simulink model "test_current_limiter"  (R2025b)
settings: Solver=ode23  StartTime=0.0  StopTime=10.0  RelTol=1e-3
StopFcn:
  | Simulink.sdi.view;
  | Simulink.sdi.loadView('view_test_current_limiter');
libraries: fl_lib x6, nesl_utility x3, arsenal x1, ee_lib x1
settings Model: Creator=ggandolfi  LastModifiedBy=upattacini
settings DataIOCC: SaveOutput=off  DSMLogging=off  SaveTime=off  ReturnWorkspaceOutputs=off

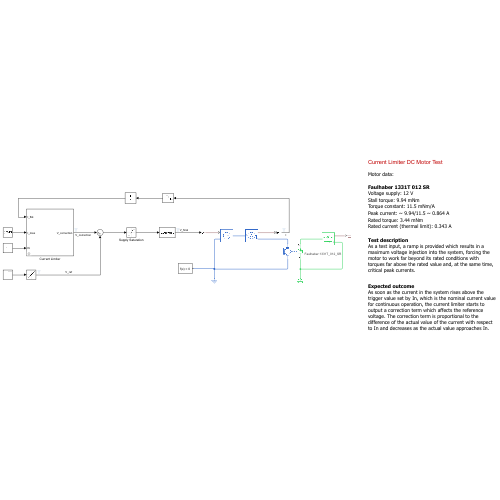
[thumbnail: Simulink's stored preview of the top-level diagram]
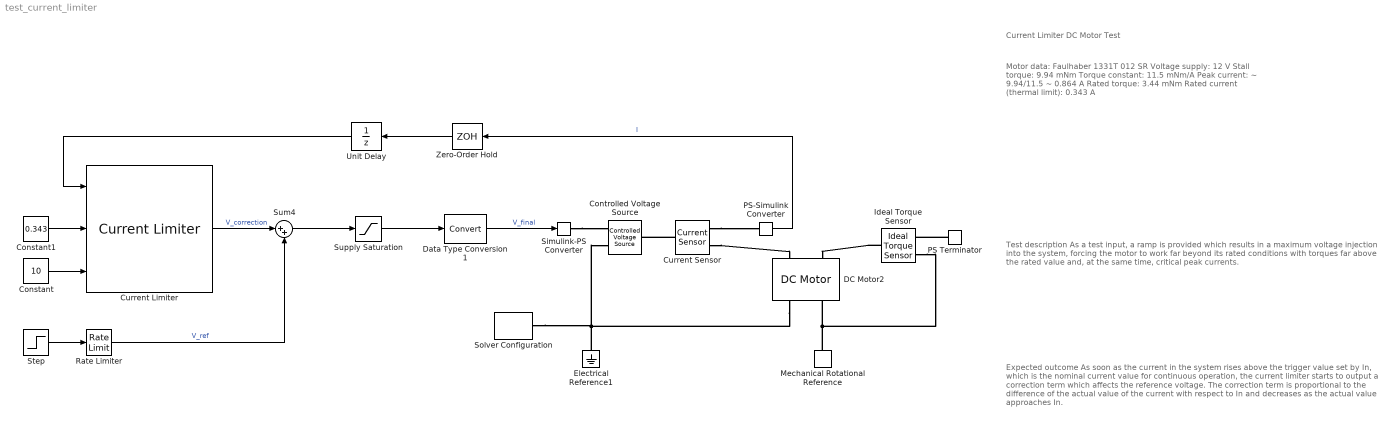
== system test_current_limiter ==
  note: Motor data:
      |
      | Faulhaber 1331T 012 SR
      | Voltage supply: 12 V
      | Stall torque: 9.94 mNm
      | Torque constant: 11.5 mNm/A
      | Peak current: ~ 9.94/11.5 ~ 0.864 A
      | Rated torque: 3.44 mNm
      | Rated current (thermal limit): 0.343 A
  note: Current Limiter DC Motor Test
  note: Test description
      | As a test input, a ramp is provided which results in a maximum voltage injection into the system, forcing the motor to work far beyond its rated conditions with torques far above the rated value and, at the same time, critical peak currents.
  note: Expected outcome
      | As soon as the current in the system rises above the trigger value set by In, which is the nominal current value for continuous operation, the current limiter starts to output a correction term which affects the reference voltage. The correction term is proportional to the difference of the actual value of the current with respect to In and decreases as the actual value approaches In.
  Constant : Constant  Value=10
  Constant1 : Constant  Value=0.343
  Controlled Voltage Source : fl_lib/Electrical/Electrical Sources/Controlled Voltage Source
  Current Limiter : arsenal/Signal Conditioning/Current Limiter  Ts=0.00005  I_max_gain=0.1  Discrete_time_integrator_gain=1.0
      settings: SourceProductName=MESH Arsenal
  Current Sensor : fl_lib/Electrical/Electrical Sensors/Current Sensor
  DC Motor2 : ee_lib/Electromechanical/Brushed Motors/DC Motor  PartSpecification="{\"CollectionId\":\"SimscapeElectrical\",\"DatasetId\":\"Faulhaber|1331T_012_SR|simscape.electrical.dcMotor\",\"DisplayName\":\"Faulhaber:1331T_012_SR\"}"  field_option=ee.enum.field_option.pm  Rf=100 % Parameter not set Ohm  Lf=1 % Parameter not set H  Laf=0.15 % Parameter not set H  If0=0 % Parameter not set A  parameterization=ee.enum.dcparam_option.torque_speed  Ra=13.7 % Datasheet derived Ohm  La=0.31 % Datasheet derived mH  emf_or_torque=ee.enum.emf_or_torque.ki  Kv=1.2 % Datasheet derived mV/rpm  Ki=11.5 % Parameter estimated mN*m/A  T_stall=9.94 m*mN  w_max=9910 rpm  w_rated=15000 % Parameter not set rpm  P_rated=0.08 % Parameter not set W  V_rated=10.5 V  lam_param=ee.enum.lam_param.current  i_noload=0.0105 % Datasheet derived A  V_i_noload=12 % Datasheet derived V  J=0.67 % Datasheet derived g*cm^2  lam=0 % % Parameter not set mN*m/(rad/s)  speed0=0 % Parameter not set rpm  alpha=3.93e-3 % Parameter not set 1/K  Tmeas=25 % Parameter not set degC  thermal_mass=27 % Parameter estimated J/K  initial_temperature=27 % Parameter not set degC
      settings: AttributesFormatString=Faulhaber:1331T_012_SR
  Data Type Conversion1 : DataTypeConversion  SaturateOnIntegerOverflow=off  RndMeth=Floor
  Electrical Reference1 : fl_lib/Electrical/Electrical Elements/Electrical Reference
  Ideal Torque Sensor : fl_lib/Mechanical/Mechanical Sensors/Ideal Torque Sensor
  Mechanical Rotational Reference : fl_lib/Mechanical/Rotational Elements/Mechanical Rotational Reference
  PS Terminator : fl_lib/Physical Signals/Sinks/PS Terminator
  PS-Simulink Converter : nesl_utility/PS-Simulink Converter  PhysicalDomain=network_engine_domain  SubClassName=ps_output  LeftPortType=input  RightPortType=output  PseudoPeriodic=off  Frequencies=[]  VectorFormat=inherit  Unit=A  AffineConversion=off
  Rate Limiter : RateLimiter  RisingSlewLimit=5  SampleTimeMode=inherited
  Simulink-PS Converter : nesl_utility/Simulink-PS Converter  PhysicalDomain=network_engine_domain  SubClassName=ps_input  LeftPortType=input  RightPortType=output  PseudoPeriodic=off  Frequencies=[]  NoiseDistribution=none  NoiseParameters=[]  Unit=V  AffineConversion=off  FilteringAndDerivatives=provide  SimscapeFilterOrder=1  InputFilterTimeConstant=0.001  UdotUserProvided=0
  Solver Configuration : nesl_utility/Solver Configuration  PhysicalDomain=network_engine_domain  SubClassName=solver  LeftPortType=input  RightPortType=generic  Tones=[]  Harmonics=[]  SimulateNoise=off  Profile=off  UseLocalSampling=off  EnableSwitchedLinearOptims=on  FrequencyDomain=off  UseCCode=off  RelTol=0.001  AbsTol=0.001  MinStep=1e-09  ToWorkspace=off  RevertToSquareIcSolve=off  NumHomotopyIterations=100  PhasorMode=off  PhasorModeNumHarmonics=1  ConsistencySolver=NEWTON_XTOL_AFTER_FTOL  IndexReductionMethod=DerivativeReplacement  DoDC=off  ResidualTolerance=1e-09  ConsistencyTolSource=GLOBAL  ConsistencyAbsTol=0.001  ConsistencyRelTol=0.001  ConsistencyTolFactor=0.001  UseLocalSolver=off  LocalSolverChoice=NE_BACKWARD_EULER_ADVANCER  ResolveIndetEquations=on  FunctionEvalNumThread=1  LocalSolverSampleTime=0.001  DoFixedCost=off  MaxNonlinIter=3  MaxModeIter=2  ComputeImpulses=off  ImpulseIterations=2  LinearAlgebra=auto  LinearAlgebraNumThread=0  EquationFormulation=NE_TIME_EF  DelaysMemoryBudget=1024  AutomaticFiltering=on  FilteringTimeConstant=0.001  PartitionStorageMethod=AS_NEEDED  PartitionMemoryBudget=1024  PartitionMethod=ROBUST  MultibodyUseLocalSolver=off  MultibodyLocalSolverChoice=ODE1  MultibodyLocalSolverSampleTime=0.001
  Step : Step  Time=0.5  After=10  SampleTime=5E-5
  Sum4 : Sum  Inputs=|++
  Supply Saturation : Saturate  UpperLimit=12  LowerLimit=-12
  Unit Delay : UnitDelay  SampleTime=5E-5  HasFrameUpgradeWarning=on
  Zero-Order Hold : ZeroOrderHold  SampleTime=5E-5
  wires:
  Constant/1 -> Current Limiter/3
  Constant1/1 -> Current Limiter/2
  Rate Limiter/1 -> Sum4/2  "V_ref"
  Current Limiter/1 -> Sum4/1  "V_correction"
  Supply Saturation/1 -> Data Type Conversion1/1
  Data Type Conversion1/1 -> Simulink-PS Converter/1  "V_final"
  Sum4/1 -> Supply Saturation/1
  PS-Simulink Converter/1 -> Zero-Order Hold/1  "I"
  Unit Delay/1 -> Current Limiter/1
  Zero-Order Hold/1 -> Unit Delay/1
  Step/1 -> Rate Limiter/1
  connections:
  Simulink-PS Converter/RConn1 -- Controlled Voltage Source/RConn1
  Electrical Reference1/LConn1 -- Solver Configuration/RConn1 -- Controlled Voltage Source/RConn2 -- DC Motor2/RConn1
  Current Sensor/LConn1 -- Controlled Voltage Source/LConn1
  Current Sensor/RConn2 -- DC Motor2/LConn1
  Current Sensor/RConn1 -- PS-Simulink Converter/LConn1
  Mechanical Rotational Reference/LConn1 -- Ideal Torque Sensor/RConn1 -- DC Motor2/RConn2
  Ideal Torque Sensor/LConn1 -- DC Motor2/LConn2
  PS Terminator/LConn1 -- Ideal Torque Sensor/RConn2
